simulink model "Bruening_4t_showshuffle"  (R2015a)
settings: Solver=ode4  SolverMode=MultiTasking  StartTime=0.0  StopTime=inf  FixedStep=BKIN_STEP_TIME  RelTol=1e-3
StartFcn:
  |  warndlg('Dexterit-E models cannot run under simulation. Please compile your model and run it from within Dexterit-E.');set_param(bdroot,'SimulationCommand','stop')
model workspace (MAT data in the model file):
  BKIN_STEP_TIME = 0.00025
  col_x = 1
  col_y = 2
  E_TARGET_ON = 3
  E_HOLD_AT_TARGET = 5
  LOGICAL_RADIUS = 4
  START_TARGET_COL = 1
  END_TARGET_COL = 2
  ROTATION_CENTER = 5
  WAIT_AT_1stTARGET_COL = 7
  MAXREACHTIME_COL = 8
  DELAY_POSTTRIAL_COL = 9
  E_STAY_CENTER = 2
  VISUAL_RADIUS = 3
  COLOR = 5
  ALTCOLOR = 6
  STROKECOLOUR = 7
  STROKEWIDTH = 9
  TARGET_EGG = 6
  LABEL_TEXT = 12
  LABEL_COLOUR = 13
  LABEL_HEIGHT = 14
  TEXT_DISPLAY_TARGET = 10
  ALTSTROKECOLOUR = 8
  SEGMENT_COUNT = 11
  E_TARGET_MISS = 6
  END_X = 10
  END_Y = 11
  E_LEFT_RING = 4
  E_START_BLOCK = 10
  BKIN_KINEMATIC_FRAME_SIZE = 400
  E_NO_EVENT = 1
  TARGET_IN_USE = 3
  R_PROB = 4
  E_R_TARG1 = 7
  E_M_TARG1 = 12
  E_R_TARG2 = 8
  E_M_TARG2 = 13
  E_R_TARG3 = 9
  E_M_TARG3 = 14
  E_R_TARG4 = 11
  E_M_TARG4 = 15
  WAIT_TIME = 12
  TONE_DURATION = 13
  FLASH_INTER = 14
  FLASH_NUM = 15
  BREAK_T1 = 16
  BREAK_T2 = 17
  ALTVISUAL_RADIUS = 15
  ALTCOLOR2 = 16
undefined symbols (not defined in the file or in its folder): slselsubs
libraries: Video x15, simulink x12, xpcrtudplib x12, xpcutilitieslib x10, xpcobsoletelib x8, ethercat x2, General x2, slrtlib x2, KINARM_general x1
(part 4 of 6)

== stateflow chart Bruening_4t_showshuffle/Trial_Control ==
  settings: sampleTime=0.001
  state Main_Trial
    state FirstTargetOn/
      // Turn on first target, set loading conditions, enable data logging, wait for specified delay or until hand-is-in-target
      targetA_row = Trial_Protocol[START_TARGET_COL];
      targetA_state=targetA_var;
      targetBlock_state = targetBlock_var;
      targetC_state = 0;
      targetL1_state = 0;
      targetL2_state = 0;
    state NewBlock/
      //Change color of home circle on first trial of a block
      event_code = E_START_BLOCK;
      targetRest_state = 0;
      targetA_var = 2;
      targetBlock_var = 1;
    state NotFirstTrial/
      targetRest_state = 0;
      targetA_var = 1;
      targetBlock_var = 0;
    state StayAtFirstTarget/
      // change the first target state (e.g. colour), log an event, wait for specified period of time.  Hand must STAY in target for specified time.
      logging_enable = 1;
      event_code=E_STAY_CENTER;
      targetA_state=targetA_var;
      tickCount =Trial_Protocol[WAIT_AT_1stTARGET_COL] + getRandomValue();
      in_target = 0;
      last_low_vel = 0;
    state Show2ndTarget/
      // Turn on second target, log an event, wait until hand-is-in-target or wait for specified delay
      cursor_feedback = 0;
      in_target = 0;
      n_low_vel = 0;
      event_code=E_TARGET_ON;
      targetSS_row = Trial_Protocol[TARGET_IN_USE];
      targetD_row = 4;
      targetE_row = 5;
      targetF_row = 6;
      targetK_row = 7;
      targetSS_state = 1;
      targetA_state = 0;
      targetBlock_state = 0;
      tickCount =Trial_Protocol[MAXREACHTIME_COL];
      during: n_low_vel1 = vel_check(hand_vel, n_low_vel)
      during: in_target  = intarget_check(hand_pos, center_pos, current_tp_index)
    state EndOfTrial/
      // Wait for a specified period of time
      flash = 0;
      tickCount =Trial_Protocol[DELAY_POSTTRIAL_COL];
      breakT1 = Trial_Protocol[BREAK_T1];
      breakT2 = Trial_Protocol[BREAK_T2];
      breakYN = getBreak(trialnum, breakT1, breakT2);
      targetD_state = 0;
      targetE_state = 0;
      targetF_state= 0;
      targetK_state = 0;
      targetL1_state = 0;
      targetL2_state = 0;
      in_target = 0;
      cursor_feedback = 1;
    state TargetMiss/
      target
      targetSS_state = 0;
      targetL2_state = 1;
      event_code = E_TARGET_MISS
      tone_frequency = 700;
    state HandExcursion/
      // When leaving ring, see if subj hit target
      t_id = target_index;
      maxR = 10;
      r_prob = Trial_Protocol[R_PROB];
      [reward, score_ret, hand_angle,angle_index] = getReward(hand_pos, t_id, center_pos,maxR,current_tp_index,r_prob)
      event_code = E_LEFT_RING; // need to be defined in param table
      targetC_state = getTS(block_index);
      tickCount =250;
      flash = 0;
      tone_duration = Trial_Protocol[TONE_DURATION];
      flash_interval = Trial_Protocol[FLASH_INTER];
      flash_num = Trial_Protocol[FLASH_NUM];
    state GetReward_Target_1/
      // When the subject hits the ring
      targetSS_state = 0;
      targetD_state = 2;
      targetL1_state = 1;
      event_code=E_R_TARG1;
      tone_frequency = 4186.01;
      e_Play_Tone;
    state GetReward_Target_2/
      // when the subject hits the ring
      targetSS_state = 0;
      targetE_state = 2;
      targetL1_state = 1;
      event_code=E_R_TARG2;
      tone_frequency = 4186.01;
      e_Play_Tone;
    state GetReward_Target_4/
      // when the subject hits the ring
      targetSS_state = 0;
      targetK_state = 2;
      targetL1_state = 1;
      event_code=E_R_TARG4;
      tone_frequency = 4186.01;
      e_Play_Tone;
    state GetReward_Target_3/
      // when the subject hits the ring
      targetSS_state = 0;
      targetF_state = 2;
      targetL1_state = 1;
      event_code=E_R_TARG3;
      tone_frequency = 4186.01;
      e_Play_Tone;
    state GetReward_Target_5/
      // When the subject hits the ring
      tone_frequency = 4698.63;
      e_Play_Tone;
    state GetReward_Target_8/
      // When the subject hits the ring
      tone_frequency = 4698.63;
      e_Play_Tone;
    state GetReward_Target_6/
      // When the subject hits the ring
      tone_frequency = 4698.63;
      e_Play_Tone;
    state GetReward_Target_7/
      // When the subject hits the ring
      tone_frequency = 4698.63;
      e_Play_Tone;
    state Flash_Target_1_1/
      // flash the target off
      targetD_state = 1;
      flash = flash+1;
    state Flash_Target_3_1/
      // flash the target off
      targetF_state = 1;
      flash = flash+1;
    state Flash_Target_2_1/
      // flash the target off
      targetE_state = 1;
      flash = flash+1;
    state Flash_Target_4_1/
      // flash the target off
      targetK_state = 1;
      flash = flash+1;
    state Flash_Target_4_2/
      // flash the target on
      targetK_state = 2;
    state Flash_Target_1_2/
      // flash the target on
      targetD_state = 2;
    state Flash_Target_2_2/
      // flash the target on
      targetE_state = 2;
    state Flash_Target_3_2/
      // flash the target on
      targetF_state = 2;
    state MissReward_Target_1/
      // when the subject hits the ring
      targetSS_state = 0;
      targetD_state = 3;
      event_code=E_M_TARG1;
    state MissReward_Target_2/
      // when the subject hits the ring
      targetSS_state = 0;
      targetE_state = 3;
      event_code=E_M_TARG2;
    state MissReward_Target_3/
      // when the subject hits the ring
      targetSS_state = 0;
      targetF_state = 3;
      event_code=E_M_TARG3;
    state MissReward_Target_4/
      // when the subject hits the ring
      targetSS_state = 0;
      targetK_state = 3;
      event_code=E_M_TARG4;
    NewBlock -> FirstTargetOn : after(150,e_clk)/
    NotFirstTrial -> FirstTargetOn
    FirstTargetOn -> StayAtFirstTarget : [HandInTarget[targetA_row]==1]
    StayAtFirstTarget -> FirstTargetOn [order 2] : [HandInTarget[targetA_row]==0]
    StayAtFirstTarget -> Show2ndTarget [order 1] : after(tickCount, e_clk)/
        |
        | // apply the new rotation amount now (i.e. wait until the subject is in the starting target before applying a new
        | // rotation, so that they do not see the hand feedback jump/change when a new rotation is applied)
        | // have this event occur on this transition, rather than in the "StayAtFirstTarget" state to ensure that the subject
        | // is really starting the trial.  Could have put this event in the "Show2ndTarget" state instead.
    Show2ndTarget -> HandExcursion [order 2] : [in_target == 1]
    Show2ndTarget -> EndOfTrial [order 1] : after(tickCount, e_clk)/
    TargetMiss -> EndOfTrial : after(250,e_clk)/
    HandExcursion -> TargetMiss [order 9] : [angle_index == 0 && reward ==0]
    HandExcursion -> GetReward_Target_1 [order 8] : [reward == maxR && current_tp_index == 1]
    HandExcursion -> MissReward_Target_4 [order 1] : [reward == 0 && angle_index == 4]
    HandExcursion -> GetReward_Target_4 [order 2] : [reward == maxR && current_tp_index == 4]
    HandExcursion -> MissReward_Target_1 [order 7] : [reward == 0 && angle_index == 1]
    HandExcursion -> GetReward_Target_2 [order 6] : [reward == maxR && current_tp_index == 2]
    HandExcursion -> MissReward_Target_2 [order 5] : [reward == 0 && angle_index == 2]
    HandExcursion -> GetReward_Target_3 [order 4] : [reward == maxR && current_tp_index == 3]
    HandExcursion -> MissReward_Target_3 [order 3] : [reward == 0 && angle_index == 3]
    GetReward_Target_2 -> GetReward_Target_6 : after(tone_duration+50, e_clk)/
    GetReward_Target_1 -> GetReward_Target_5 : after(tone_duration+50, e_clk)/
    GetReward_Target_4 -> GetReward_Target_8 : after(tone_duration+50, e_clk)/
    GetReward_Target_5 -> Flash_Target_1_1 : after(flash_interval, e_clk)/
    GetReward_Target_3 -> GetReward_Target_7 : after(tone_duration+50, e_clk)/
    GetReward_Target_7 -> Flash_Target_3_1 : after(flash_interval, e_clk)/
    GetReward_Target_8 -> Flash_Target_4_1 : after(flash_interval, e_clk)/
    GetReward_Target_6 -> Flash_Target_2_1 : after(flash_interval, e_clk)/
    Flash_Target_1_2 -> Flash_Target_1_1 : after(flash_interval, e_clk)/
    Flash_Target_1_1 -> Flash_Target_1_2 [order 2] : [flash <= flash_num && after(flash_interval, e_clk)]
    Flash_Target_4_1 -> Flash_Target_4_2 [order 2] : [flash <= flash_num && after(flash_interval, e_clk)]
    Flash_Target_3_2 -> Flash_Target_3_1 : after(flash_interval, e_clk)/
    Flash_Target_3_1 -> Flash_Target_3_2 [order 2] : [flash <= flash_num && after(flash_interval, e_clk)]
    Flash_Target_2_2 -> Flash_Target_2_1 : after(flash_interval, e_clk)/
    Flash_Target_2_1 -> Flash_Target_2_2 [order 2] : [flash <= flash_num && after(flash_interval, e_clk)]
    Flash_Target_4_2 -> Flash_Target_4_1 : after(flash_interval, e_clk)/
  state Initialize/
    // Turn off both targets, set hand_feedback on
    cursor_feedback = 1;
    targetA_state=0;
    targetB_state=1;
    targetB_row = 2;
    targetC_state = 0;
    targetC_row = 3;
    targetD_state =  0;
    targetD_row = 4;
    targetE_state = 0;
    targetE_row = 5;
    targetF_state = 0;
    targetF_row = 6;
    targetK_state = 0;
    targetK_row = 7;
    targetG_state = 1;
    targetG_row = 8;
    targetH_state = 1;
    targetH_row = 9;
    targetI_state = 1;
    targetI_row = 10;
    targetJ_state = 1;
    targetJ_row = 11;
    targetSS_state = 0;
    targetCScore_state = 1;
    targetCScore_row = 12;
    targetBlock_row = 13;
    targetBlock_state = 0;
    targetRest_row = 14;
    targetRest_state = 0;
    targetL1_state = 0;
    targetL1_row = 15;
    targetL2_state = 0;
    targetL2_row = 16;
    in_target = 0;
    //score_ret = 0;
  state Inter_Trial_State/
    // send e_Trial_End event
    e_Trial_End;
    // turn off both targets
    // stop data logging
    event_code=0;
    targetA_state=0;
    logging_enable = 0;
  state Last_Trial_State/
    // send e_Trial_End event
    e_Trial_End;
    // turn off both targets
    // stop data logging
    event_code=0;
    targetA_state=0;
    logging_enable = 0;
    tickCount = Trial_Protocol[WAIT_TIME];
    targetRest_state = 1;
  (junction 148) -> NewBlock [order 1] : [trialnum==19]
  (default) -> Initialize
  (junction 148) -> NotFirstTrial [order 2] : [isTrialOne==0 || isTrialOne == 1]
  Initialize -> (junction 148)
  Inter_Trial_State -> (junction 148)
  Last_Trial_State -> (junction 148) : after(tickCount, e_clk)/
  Main_Trial -> Inter_Trial_State : e_ExitTrialNow/
      | // if e_ExitTrialNow event occurs...
      | tickCount=1;
  (junction 229) -> Inter_Trial_State [order 1] : [breakYN == 0]
  (junction 229) -> Last_Trial_State [order 2] : [breakYN == 1]
  EndOfTrial -> (junction 229) : after(tickCount, e_clk)/
  (junction 136) -> EndOfTrial : after(tickCount, e_clk)/
  Flash_Target_1_1 -> (junction 136) [order 1]
  Flash_Target_3_1 -> (junction 136) [order 1]
  Flash_Target_2_1 -> (junction 136) [order 1]
  Flash_Target_4_1 -> (junction 136) [order 1]
  MissReward_Target_1 -> (junction 136)
  MissReward_Target_2 -> (junction 136)
  MissReward_Target_3 -> (junction 136)
  MissReward_Target_4 -> (junction 136)
  data: increment function_output double; hand_vel function_input double size=[1,2]; n_low_vel function_input double; n_low_vel1 function_output double; hand_pos function_input double size=[1,2]; in_target function_output double; center_pos function_input double size=[1,2]; current_tp_index function_input double; hand_pos function_input double size=[1,2]; target_index function_input double size=[1,3]; reward function_output double; score_ret function_output double; center_pos function_input double size=[1,2]; hand_angle function_output double; maxR function_input double; current_tp_index function_input double; angle_index function_output double; r_prob function_input double; block_index function_input double; ShowTS function_output double; trialnum function_input double; breakT1 function_input double; breakYN function_output double; breakT2 function_input double; logging_enable output boolean; event_code output uint16 [0..] =0; Trial_Protocol input double; cur_time input uint32 size=1; HandInTarget input double; targetA_row output [1..32]; targetA_state output double; targetB_row output double; targetB_state output double; tickCount local double; targetC_row output double; targetC_state output double; targetD_row output double; targetD_state output double; Target_Table local double; hand_pos input double size=[1,2]; target_index input double; center_pos input double size=[1,2]; isTrialOne input double; targetE_row output double; targetE_state output double; targetF_row output double; targetF_state output double; targetG_row output double; targetG_state output double; targetH_row output double; targetH_state output double; targetI_row output double; targetI_state output double; targetA_var local double =0; targetCScore_row output double; targetCScore_state output double; targetBlock_row output double; targetBlock_state output double; hand_angle output double; t_id output double size=[1,3]; score_ret output double; reward output double; maxR local double; tone_frequency output double; targetBlock_var local double; targetJ_row output double; targetJ_state output double; targetK_row output double; targetK_state output double; target input; midR local double; angle_index output double; current_tp_index input; targetSS_row output double; targetSS_state output double; r_prob local double; trialnum input; lastrial local double; isLastT local double; targetRest_row output double; targetRest_state output double; tone_duration output int32; waitime local double; breakT1 local int32; breakT2 local int32; breakYN local double; flash local int32; flash_interval local int32; flash_num local int32; stepindex local double; block_index input; targetL1_row output double; targetL1_state output double; targetL2_row output double; targetL2_state output double; in_target local double; hand_vel input double size=[1,2]; low_vel_t output double; ct local double; last_low_vel local double; low_vel_dur output double; last_low_vel_time local double; n_low_vel1 output double; n_low_vel local double; cursor_feedback output double
  data targetA_row settings: description=index of the row currently being used in the TargetTable
  events: e_clk input RISING_EDGE_EVENT; e_ExitTrialNow input EITHER_EDGE_EVENT; e_ApplyNewRotation local EITHER_EDGE_EVENT; e_Trial_End output EITHER_EDGE_EVENT; e_Play_Tone output FUNCTION_CALL_EVENT
  function increment = getRandomValue:
    | function increment = getRandomValue()
    | 
    |  rng(randi(10^7,1));
    |  increment = 170*rand(1) - 50;
  function n_low_vel1 = vel_check(hand_vel, n_low_vel):
    | function n_low_vel1 = vel_check(hand_vel, n_low_vel)
    | 
    | vx = hand_vel(1);
    | vy = hand_vel(2);
    | 
    | v = sqrt(vx^2+vy^2);
    | 
    | if v > 0.01
    |     n_low_vel1 = n_low_vel + 1;
    | else
    |     n_low_vel1 = 0;
    | end
    | 
    | end
  function in_target = intarget_check(hand_pos, center_pos, current_tp_index):
    | function in_target = intarget_check(hand_pos, center_pos, current_tp_index)
    | % getReward function: Computes the reward at the current instant as well as
    | % updates the score for the game
    | % Variables:
    | % hand_pos--(1X2)vector denoting the x and y positions of the hand feeback
    | % target_pos-- (1X2) vector denoting the x and y positions of the target
    | % center to be found
    | % current_tp_index: the tp used in this trial
    | % Outputs:
    | % reward : scalar that contains current reward
    | % score_ret : scalar that contains the overall score upto this point
    | 
    | % hand location in global coordinated; unit : m
    | x_hand = hand_pos(1);
    | y_hand = hand_pos(2);
    | 
    | % target center in global coordinates; 
    | % target_pos comes out at cm, this converts to m.
    | x_center = center_pos(1)/100;
    | y_center = center_pos(2)/100;
    | 
    | % % Old target Locations
    | % switch current_tp_index
    | %     case 1
    | %         tx = -0.098;
    | %         ty = 0.098;
    | %     case 2
    | %         tx = -0.098;
    | %         ty = -0.098;
    | %     case 3
    | %         tx = 0.098;
    | %         ty = -0.098;
    | %     case 4
    | %         tx = 0.098;
    | %         ty = 0.098;
    | %     case 5
    | %         tx = -0.098;
    | %         ty = 0.098;
    | %     case 6
    | %         tx = -0.098;
    | %         ty = -0.098;
    | %     case 7
    | %         tx = 0.098;
    | %         ty = -0.098;
    | %     case 8
    | %         tx = 0.098;
    | %         ty = 0.098;
    | %     otherwise
    | %         tx = 0;
    | %         ty = 0;
    | % end
    | 
    | t_pos = 0.07071;
    | switch current_tp_index
    |     case 1
    |         tx = t_pos;
    |         ty = t_pos;
    |     case 5
    |         tx = t_pos;
    |         ty = t_pos;
    |     case 2
    |         tx = -t_pos;
    |         ty = t_pos;
    |     case 6
    |         tx = -t_pos;
    |         ty = t_pos;
    |     case 3
    |         tx = -t_pos;
    |         ty = -t_pos;
    |     case 7
    |         tx = -t_pos;
    |         ty = -t_pos;
    |     case 4
    |         tx = t_pos;
    |         ty = -t_pos;
    |     case 8
    |         tx = t_pos;
    |         ty = -t_pos;    
    |     otherwise
    |         tx = 0;
    |         ty = 0;
    | end
    | 
    | x_target = x_center + tx;
    | y_target = y_center + ty;
    | 
    | hand_angle = atan2d(y_hand, x_hand);
    | t_angle = atan2d(ty,tx);
    | 
    | t = [tx,ty,0];
    | h = [x_hand,y_hand,0];
    | angle_error = atan2d(norm(cross(t,h)),dot(t,h));
    | 
    | x_hs = x_hand - x_center;
    | y_hs = y_hand - y_center;
    | p_hs = sqrt(x_hs^2+y_hs^2);
    | if p_hs>0.10% && abs(angle_error)<60
    |     in_target = 1;
    | else
    |     in_target = 0;
    | end
  function [reward, score_ret, hand_angle, angle_index] = getReward(hand_pos, target_index, center_pos ,maxR, current_tp_index, r_prob):
    | function [reward, score_ret, hand_angle, angle_index] = getReward(hand_pos, target_index, center_pos ,maxR, current_tp_index, r_prob)
    | % getReward function: Computes the reward at the current instant as well as
    | % updates the score for the game
    | % Variables:
    | % hand_pos--(1X2)vector denoting the x and y positions of the hand feeback
    | % target_pos-- (1X2) vector denoting the x and y positions of the target
    | % center to be found
    | % current_tp_index: the tp used in this trial
    | % Outputs:
    | % reward : scalar that contains current reward
    | % score_ret : scalar that contains the overall score upto this point
    | 
    | persistent score;
    | max_score = maxR;
    | reward_prob = r_prob;
    | 
    | % if isTrialOne || isempty(score)
    | %     score = 0;
    | % end
    | 
    | if isempty(score) 
    |     score = 0;
    | end
    | 
    | % hand location in global coordinated; unit : m
    | x_hand = hand_pos(1);
    | y_hand = hand_pos(2);
    | 
    | % target center in global coordinates 
    | % x_target = target_pos(1)/100;
    | % y_target = target_pos(2)/100;
    | 
    | x_center = center_pos(1)/100;
    | y_center = center_pos(2)/100;
    | 
    | % shift hand and target to local coordinates
    | x_hand = x_hand - x_center;
    | y_hand = y_hand - y_center;
    | 
    | t_pos = 0.07071;
    | switch current_tp_index
    |     case 1
    |         tx = t_pos;
    |         ty = t_pos;
    |     case 5
    |         tx = t_pos;
    |         ty = t_pos;
    |     case 2
    |         tx = -t_pos;
    |         ty = t_pos;
    |     case 6
    |         tx = -t_pos;
    |         ty = t_pos;
    |     case 3
    |         tx = -t_pos;
    |         ty = -t_pos;
    |     case 7
    |         tx = -t_pos;
    |         ty = -t_pos;
    |     case 4
    |         tx = t_pos;
    |         ty = -t_pos;
    |     case 8
    |         tx = t_pos;
    |         ty = -t_pos;    
    |     otherwise
    |         tx = 0;
    |         ty = 0;
    | end
    | 
    | x_target = x_center + tx;
    | y_target = y_center + ty;
    | 
    | hand_angle = atan2d(y_hand, x_hand);
    | t_angle = atan2d(ty,tx);
    | 
    | t = [tx,ty,0];
    | h = [x_hand,y_hand,0];
    | angle_error = atan2d(norm(cross(t,h)),dot(t,h));
    | 
    | if abs(angle_error) < 45
    |     if current_tp_index<5
    |         aa = current_tp_index;
    |     else
    |         aa = current_tp_index-4;
    |     end
    |     if any(reward_prob)
    |         r = max_score;
    |     else
    |         r = 0;
    |     end
    | else
    |     aa = 0;
    |     r = 0;
    | end
    | 
    | angle_index = aa;
    | reward = r;
    | score = score + r;
    | 
    | score_ret = score;
  function ShowTS = getTS(block_index):
    | function ShowTS = getTS(block_index)
    | 
    | BT = double(block_index);
    | 
    | if BT > 1
    |     Sh = 1;
    | else
    |     Sh = 0;
    | end
    | 
    | ShowTS = Sh;
  function breakYN = getBreak (trialnum, breakT1, breakT2):
    | function breakYN = getBreak (trialnum, breakT1, breakT2)
    | Tnum = trialnum;
    | BT1 = breakT1;
    | BT2 = breakT2;
    | if Tnum == BT1
    |     BB1 = 1;
    | elseif Tnum == BT2 
    |     BB1 = 1;
    | else
    |     BB1 = 0;
    | end
    | 
    | breakYN = BB1;
    | if mod(trialnum-16,180)==0
    |     breakYN = 1;
    | else
    |     breakYN = 0;
    | end
    | 
    | end

== matlab function Bruening_4t_showshuffle/MATLAB Function ==
  data: hand_pos input; hand_vel input; Target_Table input; out_targ_index output double; center_pos output; isTrialOne output double; x_hand output; y_hand output; vx_hand output; vy_hand output; cur_trial input; cur_block input
function [out_targ_index, center_pos, isTrialOne , x_hand, y_hand, vx_hand, vy_hand] = ...
    fcn(hand_pos, hand_vel, Target_Table, cur_trial, cur_block)
%#codegen

target_col_x=1;
target_col_y=2;

circ_target = 2;

cur_trial_num = double(cur_trial);
cur_block_num = double(cur_block);
persistent targ_index
persistent new_targ
rng(randi(2^32,1),'twister')
if isempty(targ_index)
    targ_index = zeros(1,3);
end

if isempty(new_targ)
    new_targ = 0;
end

isTrialOne = 0;
r1 = rem(cur_block_num,2);
if cur_trial_num==1 && any(r1)
    isTrialOne = 1;
    new_targ = new_targ+1;
else
    new_targ = 0;
end
if new_targ == 1
    rand_targ_ind = randperm(4,3);
    targ_index = rand_targ_ind;
    
end
out_targ_index = double(targ_index);
%out_targ_index = 2;

% x-center is in units of cm from the target table
x_center = Target_Table(circ_target, target_col_x);
y_center = Target_Table(circ_target, target_col_y);

x_hand = hand_pos(1);
y_hand = hand_pos(2);

vx_hand = hand_vel(1);
vy_hand = hand_vel(2);
% 
%target_pos = [x_target, y_target];
center_pos = [x_center, y_center];

== matlab function Bruening_4t_showshuffle/displayScoreTrial ==
  data: VCODE input; VCODE_out output; score_ret input
function VCODE_out  = displayScoreTrial(VCODE, score_ret)
%#codegen

text_prefix = 'trial score: ';
endPrefix = 14 + length(text_prefix);
VCODE(15:endPrefix) = uint8(text_prefix);

max_scoreP = 10^5;
if score_ret >= max_scoreP
    score_ret = 9.99999 * max_scoreP;
end
power_vals = nan(1,5);
power10 = floor(log10(score_ret));
if score_ret == 0
    power10 = 0;
end
for i = 0:power10
    power_vals(i+1) = power10-i;
end

power_vals = power_vals(~isnan(power_vals));

for p = 1:length(power_vals);
    VCODE(endPrefix+p) = getChar(score_ret,10^(power_vals(p)));
end

VCODE_out = VCODE;
end


function cc = getChar(number, dec)
%in simulink there is no nice way to convert a number to s string
%so what we are doing here is converting a single digit to a character.
%48 is ascii for '0', so this gets the least significant digit before
%the decimal and converts to ascii.
cc = floor(mod(number / dec, 10)) + 48;
end

== matlab function Bruening_4t_showshuffle/KINARM_HandFeedbackInTarget/Embedded MATLAB InsideTarget ==
  settings: fimath=|
      | fimath(...
      | 'RoundMode', 'floor',...
      | 'OverflowMode', 'wrap',...
      | 'ProductMode', 'KeepLSB', 'ProductWordLength', 32,...
      | 'SumMode', 'KeepLSB', 'SumWordLength', 32,...
      | 'CastBeforeSum', false)
  data: handpos input size=2; target_type input; attribcol input; num_targets input; intarget output; Target_Table input
function intarget = FIsInsideTarget(handpos, target_type, attribcol, num_targets, Target_Table)
% all dimensions in m, rad
% arguments:
% handpos: x,y positions of center of target
% attribcol: columns in target table specifying target attributes.  
% Specific to Target_Type
%	circle:
%	[X0,Y0,r...,rn] where:
%	X0,Y0 : centre of circle
%	r : logical radius of circle (i.e. radius used to determine 'in' or 'out' of target)
%	rn: logical radius of other targets (e.g. 2nd, 3rd) also specified in target row.
%   Up to 4 targets can be specified in a row
% ellipse:
%	[X0,Y0,a,b,t...,an, bn, tn] where:
%	X0,Y0 : centre of ellipse
%	a,b : major, minor radii of ellipse
%	t : rotation of ellipse in degrees
%	an,bn : major, minor radii of ellipse of other targets (e.g. 2nd, 3rd) also specified in target row
%	tn : rotation of ellipse in degrees of other targets (e.g. 2nd, 3rd) also specified in target row
%   Up to 4 targets can be specified in a row


target_col_x=1;
target_col_y=2;

x=handpos(1);
y=handpos(2);

intarget = zeros(size(Target_Table,1),4);

X0 = Target_Table(:,target_col_x)*0.01;			%Target Table sizes in cm in v1.4
Y0 = Target_Table(:,target_col_y)*0.01;			%Target Table sizes in cm in v1.4

deltax=x-X0;
deltay=y-Y0;

INT_MAX=2^32-1;

if target_type==1			%circle
	for target=1:num_targets
		r = Target_Table(:,attribcol(target))*0.01;			%Target Table sizes in cm in v1.4
		% simple euclidean distance
		distance2 = deltax.^2 + deltay.^2;					%distance2 is the square of the distance
	    intarget(:,target) = (distance2 <= r.^2);
	end
elseif target_type==2		%ellipse
	for target=1:num_targets
	    a = Target_Table(:,attribcol(target*3-2))*0.01;			%Target Table sizes in cm in v1.4
	    b = Target_Table(:,attribcol(target*3-1))*0.01;			%Target Table sizes in cm in v1.4	
	    t = Target_Table(:,attribcol(target*3))*(pi / 180.0);	%Target Table angles in degrees in v1.4
		sint=sin(t);
		cost=cos(t);
		xrotate=deltax.*cost+deltay.*sint;		%location of x point in ellipse's coordinate frame
		yrotate=-deltax.*sint+deltay.*cost;		%location of y point in ellipse's coordinate frame
		m=yrotate./xrotate;						%slope of line between the (x,y) to (x0,y0) in ellipse's coordinate frame
		y2sq=1./(1./(m.*a).^2+1./b.^2);			%y2sq is y2^2, where y2 is the intersection of the ellipse and the (x,y) to (x0,y0) line
	    intarget(:,target) = (yrotate.^2 <= y2sq);
    end
elseif target_type==3       %rectangle
    for target=1:num_targets
        w = Target_Table(:,attribcol(target*3-2))*0.01;  %width (sizes in cm in v1.4)
        h = Target_Table(:,attribcol(target*3-1))*0.01;  %height (sizes in cm in v1.4)
        
        if attribcol(target*3) > 0
            t = Target_Table(:,attribcol(target*3))*(pi / 180.0);  %angle (angles in degrees in v1.4)
        else
            t = zeros(size(Target_Table, 1), 1);
        end

        sint=sin(t);
        cost=cos(t);

        xrotate=deltax.*cost + deltay.*sint;   %location of x point in rectangle's coordinate frame
        yrotate=-deltax.*sint + deltay.*cost;  %location of y point in rectangle's coordinate frame

        intarget(:,target) = abs(xrotate) <= w/2 & abs(yrotate) <= h/2;
    end
elseif target_type==4       %line
    for target=1:num_targets
        % treat the line like a rectangle of height h and width w
        % determine height (stroke width) in the same fashion as in Show_Target
        if attribcol(target*3-2) == 0                     %0 column index means stroke width of 0
            h = zeros(size(Target_Table, 1), 1);
        elseif attribcol(target*3-2) < 0                  %-ve column index means stroke width of 1mm
            h = ones(size(Target_Table, 1), 1) .* 0.001;
        else
            h = Target_Table(:,attribcol(target*3-2)) * 0.01;  %target table contains width in cm
        end
        
        ex = Target_Table(:,attribcol(target*3-1))*0.01;  %endpoint in x relative to start point (cm)
        ey = Target_Table(:,attribcol(target*3))*0.01;    %endpoint in y relative to start point (cm)
        
        w = sqrt(ex.^2 + ey.^2);                          %width (cm)
        
        % determine the vector from the line's midpoint to the hand position
        handx = deltax - ex/2;
        handy = deltay - ey/2;
        
        t = atan2(ey, ex);                                %calculate angle of the line (rads)
        sint = sin(t);
        cost = cos(t);
        
        xrotate = handx.*cost + handy.*sint;   %location of x point in rectangle's coordinate frame
        yrotate = -handx.*sint + handy.*cost;  %location of y point in rectangle's coordinate frame
 
        intarget(:,target) = abs(xrotate) <= w/2 & abs(yrotate) <= h/2;
    end
elseif target_type==5  % triangle
    for target=1:num_targets
        w = Target_Table(:,attribcol(target*4-3))*0.01;         %length (sizes in cm in v1.4)
        
        % If a height column of 0 is specified, make the triangle equilateral. Otherwise, use the
        % values for height and peak offset from the target table.
        if attribcol(target*4-2) > 0
            h = Target_Table(:,attribcol(target*4-2))*0.01;  %height (sizes in cm in v1.4)
            p = Target_Table(:,attribcol(target*4-1))*0.01;  %peak offset (sizes in cm in v1.4)
        else
            h = w.*sin(pi/3.0);
            p = zeros(size(Target_Table, 1), 1);
        end
        
        if attribcol(target*4) > 0
            t = Target_Table(:,attribcol(target*4))*(pi / 180.0);  %angle (angles in degrees in v1.4)
        else
            t = zeros(size(Target_Table, 1), 1);
        end
        
        sint = sin(t);
        cost = cos(t);
        
        xrotate = deltax.*cost + deltay.*sint;   %location of x point in triangle's coordinate frame
        yrotate = -deltax.*sint + deltay.*cost;  %location of y point in triangle's coordinate frame
        
        % Begin to find centroid of triangle relative to the point on the base beneath the peak. "Left vertex" 
        % refers to the vertex at the left end of the base, and "right vertex" to the vertex at the right end.
        n = w./2.0 + p;  % distance along base from left vertex to peak
        m = w./2.0 - p;  % distance along base from peak to right vertex

        alpha = atan2(h, n);  % angle between base and line from left vertex to peak
        beta = atan2(h, m);   % angle between base and line from right vertex to peak
        
        length1 = sqrt(h.*h + n.*n) ./ 2.0;  % half length of line from left vertex to peak
        length2 = sqrt(h.*h + m.*m) ./ 2.0;  % half length of line from right vertex to peak

        % Determine slope of line from left vertex to midpoint of line from right vertex to peak.
        slope1 = ones(size(Target_Table, 1), 1) .* INT_MAX;
        
        for i=1:size(Target_Table, 1)
            if abs(w(i) - length2(i)*cos(beta(i))) > 0.0
                slope1(i) = length2(i)*sin(beta(i)) / (w(i) - length2(i)*cos(beta(i)));
            end
        end

        % Determine slope of line from right vertex to midpoint of line from left vertex to peak.
        slope2 = ones(size(Target_Table, 1), 1) .* INT_MAX;

        for i=1:size(Target_Table, 1)
            if abs(w(i) - length1(i)*cos(alpha(i))) > 0.0
                slope2(i) = -length1(i)*sin(alpha(i)) / (w(i) - length1(i)*cos(alpha(i)));
            end
        end

        % Calculate centroid position.
        centroid_x = -(m.*slope2 + n.*slope1) ./ (slope1 - slope2);
        centroid_y = slope1.*(centroid_x + n);

        % Test if the point is under the left side of the peak.
        is_under_left = false(size(Target_Table, 1), 1);

        for i=1:size(Target_Table, 1)
            if n(i) >= 0
                is_under_left(i) = (h(i) + (h(i)/n(i)) * (xrotate(i) + centroid_x(i))) >= (yrotate(i) + centroid_y(i));
            else
                is_under_left(i) = (h(i) + (h(i)/n(i)) * (xrotate(i) + centroid_x(i))) <= (yrotate(i) + centroid_y(i));
            end
        end
        
        % Test if the point is under the right side of the peak.
        is_under_right = false(size(Target_Table, 1), 1);

        for i=1:size(Target_Table, 1)
            if m(i) >= 0
                is_under_right(i) = (h(i) - (h(i)/m(i)) * (xrotate(i) + centroid_x(i))) >= (yrotate(i) + centroid_y(i));
            else
                is_under_right(i) = (h(i) - (h(i)/m(i)) * (xrotate(i) + centroid_x(i))) <= (yrotate(i) + centroid_y(i));
            end
        end
        
        intarget(:,target) = is_under_right & ...            %under right side of peak
                             is_under_left & ...             %under left side of peak
                             (yrotate + centroid_y) >= 0.0;  %above base
    end
end

== matlab function Bruening_4t_showshuffle/KINARM_HandFeedbackInTarget/Embedded MATLAB WhichHand ==
  settings: fimath=|
      | fimath(...
      | 'RoundMode', 'floor',...
      | 'OverflowMode', 'wrap',...
      | 'ProductMode', 'KeepLSB', 'ProductWordLength', 32,...
      | 'SumMode', 'KeepLSB', 'SumWordLength', 32,...
      | 'CastBeforeSum', false)
  data: use_dominant_hand input; dominant_hand input; hand output; cursor output
function [hand, cursor] = WhichHand(use_dominant_hand, dominant_hand)

if use_dominant_hand==1				%use the dominant hand
	hand=dominant_hand;		
	cursor = 1;
else
	hand=3-dominant_hand;			%use the non-dominant hand. i.e. if dominant_hand=2, hand=1 and vice-versa
	cursor = 2;
end

== matlab function Bruening_4t_showshuffle/displayScoreTotal ==
  data: VCODE input; VCODE_out output; score_ret input
function VCODE_out  = displayScoreTotal(VCODE, score_ret)
%#codegen
text_prefix = 'total score: ';
endPrefix = 14 + length(text_prefix);
VCODE(15:endPrefix) = uint8(text_prefix);

max_scoreP = 10^5;
if score_ret >= max_scoreP
    score_ret = 9.99999 * max_scoreP;
end
power_vals = nan(1,5);
power10 = floor(log10(score_ret));
if score_ret == 0
    power10 = 0;
end
for i = 0:power10
    power_vals(i+1) = power10-i;
end

power_vals = power_vals(~isnan(power_vals));
% endPrefix = 15;
for p = 1:length(power_vals);
    VCODE(endPrefix+p) = getChar(score_ret,10^(power_vals(p)));
end

VCODE_out = VCODE;
end

function cc = getChar(number, dec)
%in simulink there is no nice way to convert a number to s string
%so what we are doing here is converting a single digit to a character.
%48 is ascii for '0', so this gets the least significant digit before
%the decimal and converts to ascii.
cc = floor(mod(number / dec, 10)) + 48;
end

== matlab function Bruening_4t_showshuffle/DataLogging/Create KINARM Data Subsystem/bitfield ==
  data: motorStatus input; bitfield output
function bitfield = buildBitField(motorStatus)

%the bits are 0=motor enabled, 1=disabled. This logic is 
%attempting to reverse that. 
lowbits = bitand(bitxor(motorStatus(1), 3), 3);
highbits = bitand(bitxor(motorStatus(2), 3), 3);

currentLimitBits = bitand(motorStatus(3), 1) + bitshift(bitand(motorStatus(4), 1), 1) + ...
     bitshift(bitand(motorStatus(5), 1), 2) +  bitshift(bitand(motorStatus(6), 1), 3);

bitfield = lowbits + bitshift(highbits, 2) + bitshift(currentLimitBits, 4);

== matlab function Bruening_4t_showshuffle/Embedded MATLAB Function ==
  settings: fimath=|
      | fimath(...
      | 'RoundMode', 'floor',...
      | 'OverflowMode', 'wrap',...
      | 'ProductMode', 'KeepLSB', 'ProductWordLength', 32,...
      | 'SumMode', 'KeepLSB', 'SumWordLength', 32,...
      | 'CastBeforeSum', false)
  data: CursorPos output; VCODES_IN input
function CursorPos   = modify_cursor_pos( VCODES_IN)
% This block supports an embeddable subset of the MATLAB language.
% See the help menu for details. 

%This block was modified by Shruthi Sukumar, May 30, 2018

VCODES = VCODES_IN;
CursorPos = VCODES(1:2,3:4);

== stateflow chart Bruening_4t_showshuffle/DataLogging/Network Transfer Subsystem/Send Control Machine ==
  state UpdatePacketQueue [parallel]
    settings: executionOrder=1
    state AddPacketToQueue/
    AddPacketToQueue -> (junction 49) : e_data_ready_strobe
        | {
        | // Prepend the data of the new packet in the queue with the packet's index,
        | // a.k.a. "tracking number".
        | packet_index++;
        | packet_queue[queue_head][0] = single(packet_index);
        | //identify the packet version
        | packet_queue[queue_head][1] = -11;
        |
        | // Copy the new packet into the packet_queue.
        | CopyInput();
        |
        | // Increment the head pointer of the packet_queue for the next packet.
        | queue_head = fmod(queue_head + 1, packet_queue_sz);
        | }
    (default) -> AddPacketToQueue
    (junction 47) -> AddPacketToQueue : {TrackQueueSize();}
    (junction 49) -> (junction 46) [order 2]
    (junction 49) -> (junction 46) [order 1] : [packet_index == max_packet_id]
        | {packet_index = 0;}
    (junction 46) -> (junction 47) [order 2]
    (junction 46) -> (junction 47) [order 1] : [ queue_head == queue_tail]
        | {queue_tail = fmod(queue_tail + 1, packet_queue_sz);}
  note: Packet Queue Versions:
      |
      | -10 - Originals
      | -11 - Added "runID" at [4]
  state CopyInput [function]
    note: A trailing zero is added for safety, as the end of a packet is denoted
        | by a zero in place of the timestamp for a data frame. If the frame size is
        | such that the packet is completely filled, this zero would not be present
        | without this explicit addition.
    (default) -> (junction 109) : { i = 0; j=5;}
    (junction 109) -> (junction 109) [order 1] : [i < KINEMATIC_LEN]
        | {
        | packet_queue[queue_head][j] = data_in[i];
        | i++; j++;
        | }
    (junction 109) -> (junction 110) [order 2] : { packet_queue[queue_head][j] = 0.0; }
  state SendControlMachine [parallel]
    settings: executionOrder=2
    state Fixed/
      resetUDP = 0;
      state Idle
        // Wait to acquire a new packet to send.
      state SendPacket/
        // copy oldest packet in packet_queue to output
        CopyOutput(queue_tail);
        data_out[2] = queue_size;
        data_out[3] = total_timeouts;
        data_out[4] = runID;
        outstanding_packet_index = data_out[0];
        e_send;
      note: DEX-3274: The send control system here has been
          | updated extensively to account for UDP stack corruption issues.
          | The main areas here that are critical are:
          | 1. e_fast_clk on each transition. This is required in order to ensure that
          | we do not try to send more than one packet in a single time step
          | 2. The UDP reset system. The UDP reset system sees when the
          | queue has grown too large and then forces the UDP port to be reset
          | to clear what is likely corrupt data in the system.
      (default) -> Idle
      (junction 376) -> Idle [order 1] : [queue_head == queue_tail]
      (junction 377) -> (junction 376)
      (junction 376) -> SendPacket [order 2] : [queue_head != queue_tail]
      (junction 378) -> (junction 377) : e_fast_clk[ack_packet_index == outstanding_packet_index]
          | { queue_tail = fmod(queue_tail + 1, packet_queue_sz); }
      Idle -> SendPacket : e_fast_clk[queue_head != queue_tail]
      SendPacket -> (junction 378) [order 2]
      SendPacket -> (junction 379) [order 1] : e_fast_clk[after(10, e_clk)]
      (junction 407) -> SendPacket [order 1] : [exam_is_running == 0]
      (junction 380) -> SendPacket : {total_timeouts++;}
      (junction 379) -> (junction 407)
      (junction 407) -> (junction 380) [order 2]
    state ResetUDPPort/
      resetUDP = 1;
    (default) -> Fixed
    Fixed -> ResetUDPPort : e_reset_UDP
    ResetUDPPort -> Fixed : after(2, e_fast_clk)
  state CopyOutput(src_index) [function]
    (default) -> (junction 115) : { i = 0; }
    (junction 115) -> (junction 115) [order 1] : [i < FULL_PACKET_SIZE - 1]
        | {
        | data_out[i] = packet_queue[src_index][i];
        | i++;
        | }
    (junction 115) -> (junction 116) [order 2]
  state TrackQueueSize [function]
    (default) -> (junction 40)
    (junction 40) -> (junction 41) [order 1] : [queue_head < queue_tail]
        | { queue_size = queue_head + packet_queue_sz - queue_tail; }
    (junction 40) -> (junction 41) [order 2] : [queue_head >= queue_tail]
        | { queue_size = queue_head - queue_tail; }
  state FixMonitor [parallel]
    settings: executionOrder=3
    state Fix/
      e_reset_UDP;
    state NoFix/
    (default) -> NoFix
    NoFix -> Fix : [queue_size > 2500]
    Fix -> NoFix : e_fast_clk[after(1000, e_clk) ]
  data: src_index function_input double; resetUDP output double =0; data_out output single size=FULL_PACKET_SIZE; data_in input single size=KINEMATIC_LEN; queue_tail local uint32 =0; queue_size output double =0; total_timeouts output double =0; packet_index local uint32 =0; ack_packet_index input uint32; max_packet_id input uint32; runID input single; packet_queue local single size=[50000 FULL_PACKET_SIZE]; packet_queue_sz local double =50000; i local int32; j local int32; KINEMATIC_LEN constant double =300; FULL_PACKET_SIZE constant double =306; queue_head local uint32 =0; outstanding_packet_index local double; exam_is_running input double
  events: e_send output FUNCTION_CALL_EVENT; e_data_ready_strobe input RISING_EDGE_EVENT; e_clk input RISING_EDGE_EVENT; e_fast_clk input EITHER_EDGE_EVENT; e_reset_UDP local FUNCTION_CALL_EVENT

== matlab function Bruening_4t_showshuffle/DataLogging/Network Transfer Subsystem/force strobe1 ==
  data: strobe input; strobe_out output
function strobe_out = fcn(strobe)
%#eml
% DEX-3234 - it turns out that if we try to send 1 kinematic packet of data
% per UDP packet then the "strobe" from the packet creating sub-system just
% stays high - i.e. always send data. The trouble is that signal is used by
% the Sending state flow diagram and in order to be used as a proper
% stateflow input event the strobe has to change. This code runs at double
% the speed of the packet creating sub system. That allows us to force the
% strobe to zero on alternate steps so that we can properly signal on a true
% strobe going to 1.
persistent counter

if isempty(counter)
    counter = 0;
end

counter = counter + 1;

if mod(counter, 2) == 0
    strobe_out = 0;
    counter = 0;
else
    strobe_out = double(strobe);
end

== matlab function Bruening_4t_showshuffle/DataLogging/Poll Force Plates/plate1/parse packet 1 ==
  data: packet input; forces output; moments output; timer output; calibration input; gain input; ain_slope input; ain_offset input; orientation input; zero_voltage input
function [forces, moments, timer] = fcn(packet, calibration, gain, ain_slope, ain_offset, orientation, zero_voltage)
    %This pulls voltages and timer infomation from the packet we got back from
    %the lab jack.
    
    voltages = zeros(1, 8);
    timers = zeros(1, 3);
    
    for n = 1:8
        bits = readUShort(packet, 13 + ((n - 1)*2));
        voltages(n) = binaryToCalibratedAnalogVoltage(bits, ain_slope, ain_offset);
    end
    
    for n = 1:3
        timers(n) = readUInt(packet, 53 + ((n - 1)*4));
    end
    
    %convert the time stamp to a time in seconds.
    timer = timers(1) / 750000.0; 
    
    %all voltages are between -2.5 to 2.5, here we are normalizeing what we read to zero.
    voltages = voltages - zero_voltage;
    voltages = voltages(1:8); % only the first 8 channels matter.
    
    %using the calibration matrix we convert the to the forces and moments
    values = calibration * (voltages / gain)';
    forces = values(1:3);
    moments = values(4:6);
    
	%reverse the Z force to get it into global coordinates.
	forces(3) = -forces(3);
	
	%considering the positions of the cables push all measures into global coordinates
    if orientation == 0
        forces(2) = -forces(2);
        moments(2) = -moments(2);
    elseif orientation == 90
        y = forces(2);
        forces(2) = -forces(1);
        forces(1) = -y;

        y = moments(2);
        moments(2) = -moments(1);
        moments(1) = -y;
	elseif orientation == 180
        forces(1) = -forces(1);        
        moments(1) = -moments(1);        
    elseif orientation == 270
        y = forces(2);
        forces(2) = forces(1);
        forces(1) = y;

		y = moments(2);
        moments(2) = moments(1);
        moments(1) = y;
    end
end

function val = readUShort(data, offset)
    p1 = uint32(data(offset));
    p2 = uint32(data(offset + 1));
    val = double(p1 + (p2 * 256));
end

function val = readUInt(data, offset)
    p1 = uint32(data(offset));
    p2 = uint32(data(offset + 1));
    p3 = uint32(data(offset + 2));
    p4 = uint32(data(offset + 3));
    val = double(p1 + (p2 * 256) + (p3 * 2^16) + (p4 * 2^24));
end

function voltage = binaryToCalibratedAnalogVoltage(bits, ain_slope, ain_offset)
    voltage = (bits * ain_slope) + ain_offset;
end

== matlab function Bruening_4t_showshuffle/DataLogging/Poll KINARM/Force Sensor Control/Force Sensor 1 Subsystem/Create timestamp ==
  data: times_in input; timestamp_out output
function timestamp_out = fcn(times_in)

persistent start_time
persistent last_time

if isempty(start_time)
   start_time = uint32(0);
end

if isempty(last_time)
    last_time = uint32(0);
end

if start_time == 0 && times_in(2) > 0
    start_time = times_in(2);
end

if times_in(2) < start_time
    start_time = -(last_time - start_time);
end

%F/T sensor clock runs at 7Khz according to the manual,
%using a 32 bit integer for this gives about 7 days before it will roll
%over. This means we need to account for roll overs in order to make
%analysis sane.
timestamp_out = double(times_in(2) - start_time) / 7000.0;
last_time = times_in(2);

== matlab function Bruening_4t_showshuffle/DataLogging/Poll KINARM/Force Sensor Control/Force Sensor 2 Subsystem/Create timestamp ==
  data: times_in input; timestamp_out output
function timestamp_out = fcn(times_in)

persistent start_time
persistent last_time

if isempty(start_time)
   start_time = uint32(0);
end

if isempty(last_time)
    last_time = uint32(0);
end

if start_time == 0 && times_in(2) > 0
    start_time = times_in(2);
end

if times_in(2) < start_time
    start_time = -(last_time - start_time);
end

%F/T sensor clock runs at 7Khz according to the manual,
%using a 32 bit integer for this gives about 7 days before it will roll
%over. This means we need to account for roll overs in order to make
%analysis sane.
timestamp_out = double(times_in(2) - start_time) / 7000.0;
last_time = times_in(2);

== matlab function Bruening_4t_showshuffle/DataLogging/Poll KINARM/PMAC Subsystem/read_pmac/DPRAM Access Subsystem/TypeCast ==
  data: u input; y output
function y = fcn(u)

% EML determines output class and size based on first usage
% for some reason the typecast is not setting it correctly, so we 
% explicitly define it first.
y = single(0);

% in order for the typecast to work, both temp and y must be 32 bit
temp = cast(u, 'uint32');
y = typecast(temp, 'single');

== matlab function Bruening_4t_showshuffle/DataLogging/Poll KINARM/PMAC Subsystem/read_pmac/Monitor_status ==
  data: status_data input; servo_counter input; robotCount input; force_scale output; plcc_version input
function force_scale = monitor_system_status(status_data, servo_counter, robotCount, plcc_version)

persistent no_update_count;
persistent last_servo_counter;

if isempty(no_update_count)
   no_update_count = 0;
end

if isempty(last_servo_counter)
    last_servo_counter = uint32(0);
end

pmac_fault_state = uint32(status_data(2));
plcc_switch = status_data(3);
force_scale = 1;

%plcc versions >1000 are custom
if plcc_version >= 6.0 && plcc_version < 1000
    %if the task is running and the servo amp counter is not
    if plcc_switch == 4.0 && last_servo_counter == servo_counter
        no_update_count = no_update_count + 1;    
        %after 5 cycles with the counter not running we should kill forces.
        if no_update_count >= 5
            force_scale = 0;
        end
    else
        no_update_count = 0;
    end
    last_servo_counter = servo_counter; 
end

%plcc versions >1000 are custom
if plcc_version >= 7.0 && plcc_version < 1000
    %if it is unilateral and the robot state is faulted then kill the forces
    if robotCount == 1 && bitand(pmac_fault_state, 1) == 1
        force_scale = 0;
    %if the system is bilateral and either robot is faulted, kill forces.
    elseif robotCount == 2 && bitand(pmac_fault_state, 3) ~= 0
        force_scale = 0;
    end
end

if plcc_version == 0
    force_scale = 0;
end
